simulink library "mylib"  (R2019b)
settings: Solver=VariableStepAuto  StartTime=0.0  StopTime=10.0  RelTol=1e-3
undefined symbols (not defined in the file or in its folder): AG, AH, AV, BCHL, BCHV, BG, BH, CG, CH, magnitude, Ts, XMW
libraries: $bdroot x28, TElib x2
(part 1 of 3)
settings Model: Creator=j3vos  LastModifiedBy=j3vos
settings DataIOCC: ReturnWorkspaceOutputs=off
settings DebuggingCC: ArithmeticOperatorsInVariantConditions=warning
settings SFSimCC: SimUseLocalCustomCode=off  CustomCodeUndefinedFunction=UseInterfaceOnly
settings RTWCC: RTWUseLocalCustomCode=off

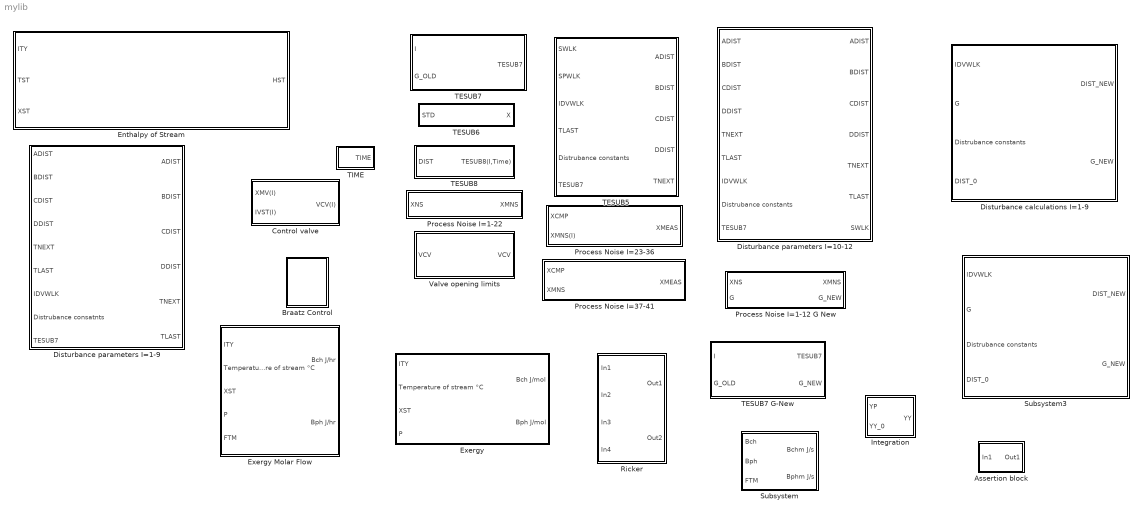
== system mylib ==
  Assertion block : Subsystem
      mask Display: color('Blue'),disp('Assertion\n Block')
  Braatz Control : Subsystem
  Control valve : Subsystem
      mask Display:
      | color('Green'), disp('Valve\nSticking');
      | color('Blue');
      | port_label('input',1,'XMV');
      | port_label('input',2,'IVST');
      | port_label('output',1,'VCV');
  Disturbance calculations I=1-9 : Subsystem
      mask Display:
      | color('Blue');
      | port_label('input',1,'IDVWLK');
      | port_label('input',2,'G');
      | port_label('input',3,'Disturbance constants');
      | port_label('input',4,'DIST_0');
      | port_label('output',1,'DIST_NEW');
      | port_label('output',2,'G_NEW');
      | color('Green'), disp('Disturbance Calculations\n I=1-9')
  Disturbance parameters I=1-9 : Subsystem
      mask Display:
      | color('Green'), disp('Disturbance parameters\n I=1-9');
      | color('Blue');
      | port_label('input',1,'ADIST');
      | port_label('input',2,'BDIST');
      | port_label('input',3,'CDIST');
      | port_label('input',4,'DDIST');
      | port_label('input',5,'TNEXT');
      | port_label('input',6,'TLAST');
      | port_label('input',7,'IDVWLK');
      | port_label('input',8,'Distrubance constants');
      | port_label('input',9,'TESUB7');
      | port_label('output',1,'ADIST');
      | port_label('output',2,'BDIST');
      | port_label('output',3,'CDIST');
      | port_label('output',4,'DDIST');
      | port_label('output',5,'TNEXT');
      | port_label('output',6,'TLAST');
  Disturbance parameters I=10-12 : Subsystem
      mask Display:
      | color('Green'), disp('Disturbance parameters\n I=10-12');
      | color('Blue');
      | port_label('input',1,'ADIST');
      | port_label('input',2,'BDIST');
      | port_label('input',3,'CDIST');
      | port_label('input',4,'DDIST');
      | port_label('input',5,'TNEXT');
      | port_label('input',6,'TLAST');
      | port_label('input',7,'IDVWLK');
      | port_label('input',8,'Distrubance constants');
      | port_label('input',9,'TESUB7');
      | port_label('output',1,'ADIST');
      | port_label('output',2,'BDIST');
      | port_label('output',3,'CDIST');
      | port_label('output',4,'DDIST');
      | port_label('output',5,'TNEXT');
      | port_label('output',6,'TLAST');
      | port_label('output',7,'SWLK');
  "Enthalpy of Stream " : Subsystem
      mask Display:
      | color('Green'), disp('TESUB1\nMolar Enthalpy of Stream\nMBtu/lb-mol');
      | color('Blue');
      | port_label('input',1,'Phase of Stream');
      | port_label('input',2,'Temperature of Stream');
      | port_label('input',3,'Composition of Stream');
      | port_label('output',1,'Enthalpy of Stream')
  Exergy : Subsystem
  Exergy Molar Flow : Subsystem
  Integration : Subsystem
  Process Noise I=1-12 G New : Subsystem
      mask Display:
      | color('Green'), disp('Process Noise');
      | color('Blue');
      | port_label('input',1,'XNS');
      | port_label('input',2,'G')
      | port_label('output',1,'XMNS');
      | port_label('output',2,'G_NEW')
  Process Noise I=1-22 : Subsystem
      mask Display:
      | color('Green'), disp('Process Noise\n I=1-22');
      | color('Blue');
      | port_label('input',1,'XNS');
      | port_label('output',1,'XMNS');
  Process Noise I=23-36 : Subsystem
      mask Display:
      | color('Green'), disp('Gas Analysis Delay\n I=23-36');
      | color('Blue');
      | port_label('input',1,'XCMP');
      | port_label('input',2,'XMNS');
      | port_label('output',1,'XMEAS');
  Process Noise I=37-41 : Subsystem
      mask Display:
      | color('Green'), disp('Product Analysis Delay\n I=37-41');
      | color('Blue');
      | port_label('input',1,'XCMP');
      | port_label('input',2,'XMNS');
      | port_label('output',1,'XMEAS');
  Ricker : Subsystem
  Subsystem : Subsystem
  Subsystem3 : Subsystem
      mask Display:
      | color('Blue');
      | port_label('input',1,'IDVWLK');
      | port_label('input',2,'G');
      | port_label('input',3,'Disturbance constants');
      | port_label('input',4,'DIST_0');
      | port_label('output',1,'DIST_NEW');
      | port_label('output',2,'G_NEW');
      | color('Green'), disp('Disturbance Calculations\n I=10-12')
  TESUB5 : Subsystem
      mask Display:
      | color('Green'), disp('TESUB5');
      | color('Blue');
      | port_label('input',1,'SWLK');
      | port_label('input',2,'SPWLK');
      | port_label('input',3,'IDVWLK');
      | port_label('input',4,'TLAST');
      | port_label('input',5,'Disturbance constants');
      | port_label('input',6,'TESUB7');
      | port_label('output',1,'ADIST');
      | port_label('output',2,'BDIST');
      | port_label('output',3,'CDIST');
      | port_label('output',4,'DDIST');
      | port_label('output',5,'TNEXT');
  TESUB6 : Subsystem
      mask Display:
      | color('Green'), disp('TESUB6');
      | color('Blue');
      | port_label('input',1,'XNS(I)');
      | port_label('output',1,'XMNS')
  TESUB7 : Subsystem
      mask Display:
      | color('Green'), port_label('output',1,'TESUB7');
      | color('Blue');
      | port_label('input',1,'I');
      | port_label('input',2,'Random number G');
  TESUB7 G-New : Subsystem
      mask Display:
      | color('Green'), port_label('output',1,'TESUB7');
      | color('Blue');
      | port_label('input',1,'I');
      | port_label('input',2,'Random number G');
  TESUB8 : Subsystem
      mask Display:
      | color('Blue');
      | port_label('input',1,'DIST');
      | color('Green'), port_label('output',1,'TESUB8(I,Time)')
  TIME : Subsystem
  Valve opening limits : Subsystem
      mask Display:
      | color('Green'), disp('Valve\nopening\nlimits');
      | color('Blue');
      | port_label('input',1,'VCV');
      | port_label('output',1,'VCV');

== system mylib/Assertion block ==
  In1 : Inport
  Data Type Conversion1 : DataTypeConversion  OutDataTypeStr=double
  Delay : Delay  DelayLength=1  InitialCondition=0
  If : If  NumInputs=2  IfExpression=u1 == 0  ElseIfExpressions=u2 == 1
  If Action Subsystem1 : Subsystem  TreatAsAtomicUnit=on
  If Action Subsystem2 : Subsystem  TreatAsAtomicUnit=on
  If Action Subsystem3 : Subsystem  TreatAsAtomicUnit=on
  Merge : Merge  Inputs=3
  Sum of Elements : Sum
  Out1 : Outport
  wires:
  If Action Subsystem2/1(Out1) -> Merge/3
  If Action Subsystem3/1(Out1) -> Merge/2
  If/1 -> If Action Subsystem1/Action
  Data Type Conversion1/1 -> Sum of Elements/1, If/1
  Sum of Elements/1 -> Delay/1, If/2
  If/3 -> If Action Subsystem2/Action
  If/2 -> If Action Subsystem3/Action
  If Action Subsystem1/1(Out1) -> Merge/1
  Delay/1 -> Sum of Elements/2
  In1/1 -> Data Type Conversion1/1
  Merge/1 -> Out1/1

== system mylib/Braatz Control ==
  P Control : Subsystem
  PI Control : Subsystem
  PI Control Setpoint : Subsystem
  Sampling interval : Subsystem
      mask Display: color('Blue'), disp('Sampling\ninterval');
  Subsystem1 : Subsystem
      mask Display: color('Blue'), disp('Valve open/close\nLimits');

== system mylib/Control valve ==
  XMV(I) : Inport
  IVST(I) : Inport  Port=2
  Delay : Delay  DelayLength=1  InitialConditionSource=Input port  InitialCondition=0
      settings: InputPortMap=u0,p4
  Subsystem : Subsystem
  Valve opening limits : $bdroot/Valve opening limits  SystemSampleTime=-1  Latency=0  AutoFrameSizeCalculation=off
  VCV(I) : Outport  VectorParamsAs1DForOutWhenUnconnected=off
  wires:
  Valve opening limits/1 -> Delay/1, VCV(I)/1
  XMV(I)/1 -> Subsystem/1(XMV(I)), Delay/2
  Delay/1 -> Subsystem/2("VCV(I) ")
  Subsystem/1(VCV(I)) -> Valve opening limits/1
  IVST(I)/1 -> Subsystem/3(IVST(I))

== system mylib/Disturbance calculations I=1-9 ==
  IDVWLK : Inport
  G : Inport  Port=2
  Distrubance constants : Inport  Port=3
  DIST_0 : Inport  Port=4
  Bus Selector : BusSelector  OutputSignals=TNEXT
  If Action Subsystem : Subsystem  TreatAsAtomicUnit=on
  If Action Subsystem1 : Subsystem  TreatAsAtomicUnit=on
  Merge : Merge
  Subsystem : Subsystem
  Subsystem1 : Subsystem
  Subsystem2 : Subsystem
  DIST_NEW : Outport  VectorParamsAs1DForOutWhenUnconnected=off
  G_NEW : Outport  Port=2  VectorParamsAs1DForOutWhenUnconnected=off
  wires:
  Subsystem2/1(G1) -> G_NEW/1
  If Action Subsystem/1(DIST_NEW) -> Merge/2
  Bus Selector/1 -> Subsystem/1(TNEXT)  "<TNEXT>"
  If Action Subsystem1/1(DIST) -> Merge/1
  DIST_0/1 -> If Action Subsystem1/1(DIST_0)
  Merge/1 -> Subsystem1/1(DIST_NEW), DIST_NEW/1
  IDVWLK/1 -> If Action Subsystem/1(IDVWLK)
  G/1 -> Subsystem2/2(G), If Action Subsystem/3(G)
  Distrubance constants/1 -> If Action Subsystem/4(Distrubance constants)
  Subsystem1/1(DIST) -> If Action Subsystem/2("DIST "), Bus Selector/1
  If Action Subsystem/2(G_NEW) -> Subsystem2/1(In2)
  Subsystem/1(if) -> If Action Subsystem1/Action
  Subsystem/2(elseif) -> If Action Subsystem/Action

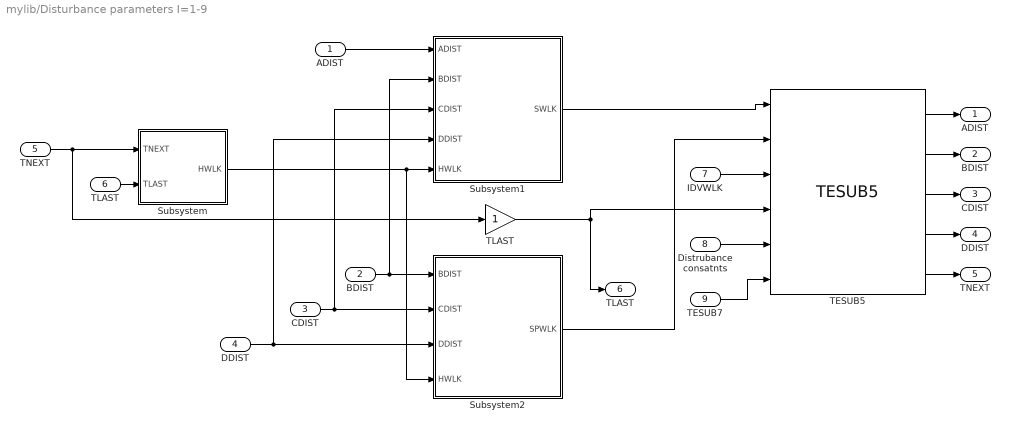
== system mylib/Disturbance parameters I=1-9 ==
  ADIST : Inport
  BDIST : Inport  Port=2
  CDIST : Inport  Port=3
  DDIST : Inport  Port=4
  TNEXT : Inport  Port=5
  TLAST : Inport  Port=6
  IDVWLK : Inport  Port=7
  Distrubance consatnts : Inport  Port=8
  TESUB7 : Inport  Port=9
  Subsystem : Subsystem
  Subsystem1 : Subsystem
  Subsystem2 : Subsystem
  TESUB5 : $bdroot/TESUB5  SystemSampleTime=-1  Latency=0  AutoFrameSizeCalculation=off
  "TLAST " : Gain
  "ADIST " : Outport  VectorParamsAs1DForOutWhenUnconnected=off
  "BDIST " : Outport  Port=2  VectorParamsAs1DForOutWhenUnconnected=off
  "CDIST " : Outport  Port=3  VectorParamsAs1DForOutWhenUnconnected=off
  "DDIST " : Outport  Port=4  VectorParamsAs1DForOutWhenUnconnected=off
  "TNEXT " : Outport  Port=5  VectorParamsAs1DForOutWhenUnconnected=off
  "TLAST  " : Outport  Port=6  VectorParamsAs1DForOutWhenUnconnected=off
  wires:
  BDIST/1 -> Subsystem2/1(BDIST), Subsystem1/2(BDIST)
  CDIST/1 -> Subsystem1/3(CDIST), Subsystem2/2(CDIST)
  DDIST/1 -> Subsystem1/4(DDIST), Subsystem2/3(DDIST)
  IDVWLK/1 -> TESUB5/3
  TNEXT/1 -> "TLAST "/1, Subsystem/1(TNEXT)
  "TLAST "/1 -> TESUB5/4, "TLAST  "/1
  TESUB5/1 -> "ADIST "/1
  TESUB5/2 -> "BDIST "/1
  TESUB5/3 -> "CDIST "/1
  TESUB5/4 -> "DDIST "/1
  TESUB5/5 -> "TNEXT "/1
  TLAST/1 -> Subsystem/2(TLAST)
  ADIST/1 -> Subsystem1/1(ADIST)
  Subsystem1/1("SWLK ") -> TESUB5/1
  Subsystem/1("HWLK ") -> Subsystem2/4(HWLK), Subsystem1/5(HWLK)
  Subsystem2/1("SPWLK ") -> TESUB5/2
  Distrubance consatnts/1 -> TESUB5/5
  TESUB7/1 -> TESUB5/6

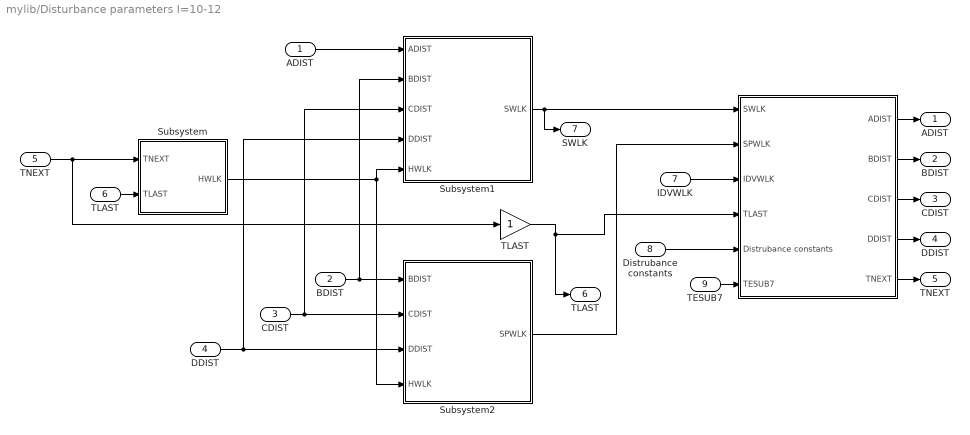
== system mylib/Disturbance parameters I=10-12 ==
  ADIST : Inport
  BDIST : Inport  Port=2
  CDIST : Inport  Port=3
  DDIST : Inport  Port=4
  TNEXT : Inport  Port=5
  TLAST : Inport  Port=6
  IDVWLK : Inport  Port=7
  Distrubance constants : Inport  Port=8
  TESUB7 : Inport  Port=9
  " " : Subsystem
  Subsystem : Subsystem
  Subsystem1 : Subsystem
  Subsystem2 : Subsystem
  "TLAST " : Gain
  "ADIST " : Outport  VectorParamsAs1DForOutWhenUnconnected=off
  "BDIST " : Outport  Port=2  VectorParamsAs1DForOutWhenUnconnected=off
  "CDIST " : Outport  Port=3  VectorParamsAs1DForOutWhenUnconnected=off
  "DDIST " : Outport  Port=4  VectorParamsAs1DForOutWhenUnconnected=off
  "TNEXT " : Outport  Port=5  VectorParamsAs1DForOutWhenUnconnected=off
  "TLAST  " : Outport  Port=6  VectorParamsAs1DForOutWhenUnconnected=off
  SWLK : Outport  Port=7  VectorParamsAs1DForOutWhenUnconnected=off
  wires:
  BDIST/1 -> Subsystem2/1(BDIST), Subsystem1/2(BDIST)
  CDIST/1 -> Subsystem1/3(CDIST), Subsystem2/2(CDIST)
  DDIST/1 -> Subsystem1/4(DDIST), Subsystem2/3(DDIST)
  IDVWLK/1 -> " "/3(IDVWLK)
  TNEXT/1 -> "TLAST "/1, Subsystem/1(TNEXT)
  "TLAST "/1 -> "TLAST  "/1, " "/4(TLAST)
  " "/1(ADIST) -> "ADIST "/1
  " "/2(BDIST) -> "BDIST "/1
  " "/3(CDIST) -> "CDIST "/1
  " "/4(DDIST) -> "DDIST "/1
  " "/5(TNEXT) -> "TNEXT "/1
  TLAST/1 -> Subsystem/2(TLAST)
  ADIST/1 -> Subsystem1/1(ADIST)
  Subsystem1/1("SWLK ") -> SWLK/1, " "/1(SWLK)
  Subsystem/1("HWLK ") -> Subsystem1/5(HWLK), Subsystem2/4(HWLK)
  Subsystem2/1("SPWLK ") -> " "/2(SPWLK)
  Distrubance constants/1 -> " "/5(Distrubance constants)
  TESUB7/1 -> " "/6(TESUB7)

== system mylib/Enthalpy of Stream  ==
  ITY : Inport
  TST : Inport  Port=2
  XST : Inport  Port=3
  Calculate Enthalpy if ITY=2 : Subsystem
  Calculate Molar Liquid Enthalpy of stream MBtu/lb-mol : Subsystem
  Calculate Molar Vapour Enthalpy of stream MBtu/lb-mol : Subsystem
  H Molar Enthalpy of stream MBtu/lb-mol : Merge  Inputs=3
  If : If  IfExpression=u1 == 0  ElseIfExpressions=u1 == 2
  If Action Subsystem : Subsystem  TreatAsAtomicUnit=on
  If Action Subsystem1 : Subsystem  TreatAsAtomicUnit=on
  If Action Subsystem2 : Subsystem  TreatAsAtomicUnit=on
  HST : Outport  VectorParamsAs1DForOutWhenUnconnected=off
  wires:
  Calculate Molar Vapour Enthalpy of stream MBtu/lb-mol/1(H) -> Calculate Enthalpy if ITY=2/2(H), If Action Subsystem2/1(In1)
  If/2 -> If Action Subsystem1/Action
  TST/1 -> Calculate Molar Liquid Enthalpy of stream MBtu/lb-mol/1(T), Calculate Enthalpy if ITY=2/1(T), Calculate Molar Vapour Enthalpy of stream MBtu/lb-mol/1(T)
  XST/1 -> Calculate Molar Vapour Enthalpy of stream MBtu/lb-mol/2(XST(I,1)), Calculate Molar Liquid Enthalpy of stream MBtu/lb-mol/2(XST(I,1))
  If Action Subsystem1/1(Out1) -> H Molar Enthalpy of stream MBtu/lb-mol/2
  If/1 -> If Action Subsystem/Action
  Calculate Enthalpy if ITY=2/1("H ") -> If Action Subsystem1/1(In1)
  ITY/1 -> If/1
  Calculate Molar Liquid Enthalpy of stream MBtu/lb-mol/1(H) -> If Action Subsystem/1(In1)
  If Action Subsystem2/1(Out1) -> H Molar Enthalpy of stream MBtu/lb-mol/3
  If/3 -> If Action Subsystem2/Action
  If Action Subsystem/1(Out1) -> H Molar Enthalpy of stream MBtu/lb-mol/1
  H Molar Enthalpy of stream MBtu/lb-mol/1 -> HST/1

== system mylib/Exergy ==
  ITY : Inport
  Temperature of stream °C : Inport  Port=2
  XST : Inport  Port=3
  P : Inport  Port=4
  Gain : Gain  Gain=2.32601*10e6
  Subsystem : Subsystem
  Subsystem2 : Subsystem
  Bch J/mol : Outport  VectorParamsAs1DForOutWhenUnconnected=off
  Bph J/mol : Outport  Port=2  VectorParamsAs1DForOutWhenUnconnected=off
  wires:
  ITY/1 -> Subsystem/1(ITY), Subsystem2/1(ITY)
  Temperature of stream °C/1 -> Subsystem2/2(Temperature of stream °C)
  XST/1 -> Subsystem/2("XST "), Subsystem2/3(XST)
  P/1 -> Subsystem2/4(P)
  Subsystem2/1(Bph MBtu/lb-mol) -> Gain/1
  Subsystem/1(Bch J/mol) -> Bch J/mol/1
  Gain/1 -> Bph J/mol/1

== system mylib/Exergy Molar Flow ==
  ITY : Inport
  Temperature of stream °C : Inport  Port=2
  XST : Inport  Port=3
  P : Inport  Port=4
  FTM : Inport  Port=5
  Gain : Gain  Gain=2.32601*10e6
  Product : Product
  Product1 : Product
  Subsystem : Subsystem
  Subsystem2 : Subsystem
  mol : Constant  Value=453.59
  mol/h : Product
  Bch J/hr : Outport  VectorParamsAs1DForOutWhenUnconnected=off
  Bph J/hr : Outport  Port=2  VectorParamsAs1DForOutWhenUnconnected=off
  wires:
  Subsystem2/1(Bph MBtu/lb-mol) -> Gain/1
  P/1 -> Subsystem2/4(P)
  XST/1 -> Subsystem2/3(XST), Subsystem/2("XST ")
  Temperature of stream °C/1 -> Subsystem2/2(Temperature of stream °C)
  ITY/1 -> Subsystem2/1(ITY), Subsystem/1(ITY)
  mol/1 -> mol/h/1
  FTM/1 -> mol/h/2
  mol/h/1 -> Product1/2, Product/2
  Subsystem/1(Bch kJ/mol) -> Product/1
  Product/1 -> Bch J/hr/1
  Gain/1 -> Product1/1
  Product1/1 -> Bph J/hr/1

== system mylib/Integration ==
  YP : Inport
  YY_0 : Inport  Port=2
  Display{,1..3} (4 alike) : Display
  Integrator : Integrator  InitialConditionSource=external
  Subsystem : Subsystem
  YY : Outport
  wires:
  YY_0/1 -> Integrator/2, Display3/1
  Integrator/1 -> YY/1, Display/1
  YP/1 -> Subsystem/1(In1), Display2/1
  Subsystem/1(Out1) -> Integrator/1, Display1/1

== system mylib/Process Noise I=1-12 G New ==
  XNS : Inport
  G : Inport  Port=2
  TESUB6 : Subsystem
      mask Display:
      | color('Green'), disp('TESUB6');
      | color('Blue');
      | port_label('input',1,'XNS(I)');
      | port_label('input',2,'G');
      | port_label('output',1,'XMNS');
      | port_label('output',2,'G_NEW')
  XMNS : Outport  VectorParamsAs1DForOutWhenUnconnected=off
  G_NEW : Outport  Port=2  VectorParamsAs1DForOutWhenUnconnected=off
  wires:
  XNS/1 -> TESUB6/1(STD)
  TESUB6/1(X) -> XMNS/1
  TESUB6/2(G_NEW) -> G_NEW/1
  G/1 -> TESUB6/2(G)

== system mylib/Process Noise I=1-22 ==
  XNS : Inport
  Clock : Clock
  If : If  NumInputs=2  IfExpression=u1>0 & u2==1  ShowElse=off
  If Action Subsystem : Subsystem  TreatAsAtomicUnit=on
  TESUB6 : $bdroot/TESUB6  SystemSampleTime=-1  Latency=0  AutoFrameSizeCalculation=off
  XMNS : Outport  VectorParamsAs1DForOutWhenUnconnected=off
  wires:
  [ISD] -> If/2
  If/1 -> If Action Subsystem/Action
  XNS/1 -> TESUB6/1
  Clock/1 -> If/1
  TESUB6/1 -> If Action Subsystem/1(In1)
  If Action Subsystem/1(Out1) -> XMNS/1

== system mylib/Process Noise I=23-36 ==
  XCMP : Inport
  XMNS(I) : Inport  Port=2
  Clock : Clock
  Delay : Delay  DelayLength=1  InitialConditionSource=Input port  InitialCondition=0
      settings: InputPortMap=u0,p4
  Delay1 : Delay  DelayLength=1  InitialConditionSource=Input port  InitialCondition=0
      settings: InputPortMap=u0,p4
  Gas Analysis Delay : Subsystem
  If : If  IfExpression=u1 == 0  ShowElse=off
  If Action Subsystem : Subsystem  TreatAsAtomicUnit=on
  If Action Subsystem1 : Subsystem  TreatAsAtomicUnit=on
  XMEAS : Outport  VectorParamsAs1DForOutWhenUnconnected=off
  wires:
  Delay1/1 -> XMEAS/1
  If/1 -> If Action Subsystem1/Action
  Clock/1 -> If/1
  Delay/1 -> If Action Subsystem/2(XDEL_OLD)
  If Action Subsystem1/1(Out1) -> Delay/2
  Gas Analysis Delay/1(IF(TGAS)) -> If Action Subsystem/Action
  If Action Subsystem/1(XDEL_NEW) -> Delay/1
  If Action Subsystem/2(XMEAS) -> Delay1/1
  XCMP/1 -> If Action Subsystem1/1(In1), If Action Subsystem/1(XCMP), Delay1/2
  XMNS(I)/1 -> If Action Subsystem/3(XMNS)

== system mylib/Process Noise I=37-41 ==
  XCMP : Inport
  XMNS : Inport  Port=2
  Clock : Clock
  Delay : Delay  DelayLength=1  InitialConditionSource=Input port  InitialCondition=0
      settings: InputPortMap=u0,p4
  Delay1 : Delay  DelayLength=1  InitialConditionSource=Input port  InitialCondition=0
      settings: InputPortMap=u0,p4
  Gas Analysis Delay : Subsystem
  If : If  IfExpression=u1 == 0  ShowElse=off
  If Action Subsystem : Subsystem  TreatAsAtomicUnit=on
  If Action Subsystem1 : $bdroot/Process Noise I=23-36/If Action Subsystem1  SystemSampleTime=-1  Latency=0  AutoFrameSizeCalculation=off
  XMEAS : Outport  VectorParamsAs1DForOutWhenUnconnected=off
  wires:
  Delay1/1 -> XMEAS/1
  XCMP/1 -> If Action Subsystem1/1, If Action Subsystem/1(XCMP), Delay1/2
  XMNS/1 -> If Action Subsystem/3(XMNS)
  Delay/1 -> If Action Subsystem/2(XDEL_OLD)
  If Action Subsystem/1(XDEL_NEW) -> Delay/1
  If/1 -> If Action Subsystem1/Action
  Gas Analysis Delay/1(IF(TPROD)) -> If Action Subsystem/Action
  If Action Subsystem1/1 -> Delay/2
  If Action Subsystem/2(XMEAS) -> Delay1/1
  Clock/1 -> If/1

== system mylib/Ricker ==
  In1 : Inport
  In2 : Inport  Port=2
  In3 : Inport  Port=3
  In4 : Inport  Port=4
  Discrete PI : TElib/Discrete PI  Kc=0  Ti=inf  Ts=1  x0=0  Hi=1  Lo=-1
  Vel PI : TElib/Discrete PI/Vel PI  Kc=Kc  Ti=Ti  Ts=Ts
  Out1 : Outport  VectorParamsAs1DForOutWhenUnconnected=off
  Out2 : Outport  Port=2  VectorParamsAs1DForOutWhenUnconnected=off
  wires:
  In3/1 -> Vel PI/1
  In1/1 -> Discrete PI/1
  In4/1 -> Vel PI/2
  Vel PI/1 -> Out2/1
  In2/1 -> Discrete PI/2
  Discrete PI/1 -> Out1/1

== system mylib/Subsystem ==
  Bch : Inport
  Bph : Inport  Port=2
  FTM : Inport  Port=3
  Gain : Gain  Gain=1/3600
  Gain1 : Gain  Gain=1/3600
  Product : Product
  Product1 : Product
  mol : Constant  Value=453.59
  mol/h : Product
  Bchm J/s : Outport  VectorParamsAs1DForOutWhenUnconnected=off
  Bphm J/s : Outport  Port=2  VectorParamsAs1DForOutWhenUnconnected=off
  wires:
  Gain1/1 -> Bchm J/s/1
  Gain/1 -> Bphm J/s/1
  Bch/1 -> Product/1
  mol/h/1 -> Product/2, Product1/2
  FTM/1 -> mol/h/2
  mol/1 -> mol/h/1
  Product1/1 -> Gain/1
  Product/1 -> Gain1/1
  Bph/1 -> Product1/1

== system mylib/Subsystem3 ==
  IDVWLK : Inport
  G : Inport  Port=2
  Distrubance constants : Inport  Port=3
  DIST_0 : Inport  Port=4
  Bus Selector : BusSelector  OutputSignals=TNEXT
  If Action Subsystem : Subsystem  TreatAsAtomicUnit=on
  If Action Subsystem1 : Subsystem  TreatAsAtomicUnit=on
  Merge : Merge
  Subsystem : Subsystem
  Subsystem1 : Subsystem
  Subsystem2 : Subsystem
  DIST_NEW : Outport  VectorParamsAs1DForOutWhenUnconnected=off
  G_NEW : Outport  Port=2  VectorParamsAs1DForOutWhenUnconnected=off
  wires:
  If Action Subsystem/1(DIST_NEW) -> Merge/2
  IDVWLK/1 -> If Action Subsystem/1(IDWLK)
  If Action Subsystem1/1(DIST) -> Merge/1
  Subsystem1/1(DIST) -> If Action Subsystem/2("DIST "), Bus Selector/1
  Merge/1 -> Subsystem1/1(DIST_NEW), DIST_NEW/1
  G/1 -> Subsystem2/2(G), If Action Subsystem/3(G)
  If Action Subsystem/2("G_NEW ") -> Subsystem2/1(In2)
  Subsystem2/1(G1) -> G_NEW/1
  Distrubance constants/1 -> If Action Subsystem/4(Distrubance constants)
  DIST_0/1 -> If Action Subsystem1/1(DIST_0)
  Bus Selector/1 -> Subsystem/1(TNEXT)  "<TNEXT>"
  Subsystem/1(if) -> If Action Subsystem1/Action
  Subsystem/2(elseif) -> If Action Subsystem/Action

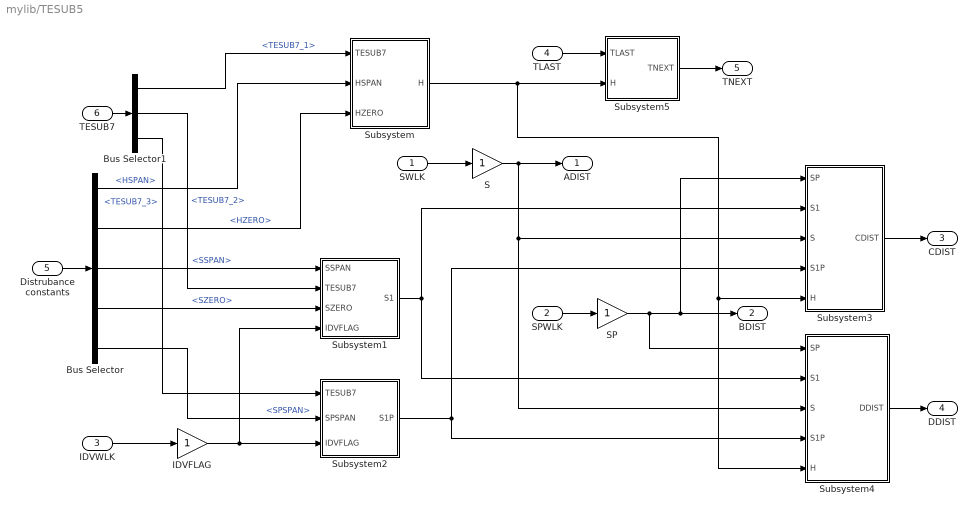
== system mylib/TESUB5 ==
  SWLK : Inport
  SPWLK : Inport  Port=2
  IDVWLK : Inport  Port=3
  TLAST : Inport  Port=4
  "Distrubance constants " : Inport  Port=5
  TESUB7 : Inport  Port=6
  Bus Selector : BusSelector  OutputSignals=HSPAN,HZERO,SSPAN,SZERO,SPSPAN
  Bus Selector1 : BusSelector  OutputSignals=TESUB7_1,TESUB7_2,TESUB7_3
  IDVFLAG : Gain
  S : Gain
  SP : Gain
  Subsystem : Subsystem
  Subsystem1 : Subsystem
  Subsystem2 : Subsystem
  Subsystem3 : Subsystem
  Subsystem4 : Subsystem
  Subsystem5 : Subsystem
  ADIST : Outport  VectorParamsAs1DForOutWhenUnconnected=off
  BDIST : Outport  Port=2  VectorParamsAs1DForOutWhenUnconnected=off
  CDIST : Outport  Port=3  VectorParamsAs1DForOutWhenUnconnected=off
  DDIST : Outport  Port=4  VectorParamsAs1DForOutWhenUnconnected=off
  TNEXT : Outport  Port=5  VectorParamsAs1DForOutWhenUnconnected=off
  wires:
  Bus Selector1/3 -> Subsystem2/1(TESUB7)  "<TESUB7_3>"
  Bus Selector1/2 -> Subsystem1/2(TESUB7)  "<TESUB7_2>"
  Bus Selector1/1 -> Subsystem/1(TESUB7)  "<TESUB7_1>"
  TESUB7/1 -> Bus Selector1/1
  IDVWLK/1 -> IDVFLAG/1
  IDVFLAG/1 -> Subsystem1/4(IDVFLAG), Subsystem2/3(IDVFLAG)
  SWLK/1 -> S/1
  SPWLK/1 -> SP/1
  S/1 -> ADIST/1, Subsystem4/3(S), Subsystem3/3(S)
  SP/1 -> Subsystem3/1(SP), BDIST/1, Subsystem4/1(SP)
  Subsystem/1("H ") -> Subsystem5/2(H), Subsystem4/5(H), Subsystem3/5(H)
  Subsystem1/1("S1 ") -> Subsystem3/2(S1), Subsystem4/2(S1)
  Subsystem2/1("S1P ") -> Subsystem3/4(S1P), Subsystem4/4(S1P)
  Subsystem3/1(CDIST) -> CDIST/1
  Subsystem4/1(DDIST) -> DDIST/1
  TLAST/1 -> Subsystem5/1(TLAST)
  Subsystem5/1(TNEXT) -> TNEXT/1
  Bus Selector/4 -> Subsystem1/3(SZERO)  "<SZERO>"
  Bus Selector/3 -> Subsystem1/1(SSPAN)  "<SSPAN>"
  Bus Selector/1 -> Subsystem/2(HSPAN)  "<HSPAN>"
  Bus Selector/5 -> Subsystem2/2(SPSPAN)  "<SPSPAN>"
  "Distrubance constants "/1 -> Bus Selector/1
  Bus Selector/2 -> Subsystem/3(HZERO)  "<HZERO>"

== system mylib/TESUB6 ==
  STD : Inport
  Constant : Constant  Value=6
  I : Constant  Value=1:12
  Product : Product
  Subtract : Sum  Inputs=+-
  TESUB7 : Subsystem
  X : Outport  VectorParamsAs1DForOutWhenUnconnected=off
  wires:
  I/1 -> TESUB7/2(I)
  [G] -> TESUB7/1(G)
  TESUB7/1(TESUB7) -> Subtract/1
  Constant/1 -> Subtract/2
  Subtract/1 -> Product/1
  Product/1 -> X/1
  STD/1 -> Product/2

== system mylib/TESUB7 ==
  I : Inport
  G_OLD : Inport  Port=2
  Constant : Constant  Value=2
  Constant1 : Constant  Value=4294967296
  Constant2 : Constant
  Divide : Product  Inputs=*/
  Divide1 : Product  Inputs=**/
  Gain : Gain  Gain=9228907
  If : If  IfExpression=u1 >=0  ElseIfExpressions=u1 <0  ShowElse=off
  If Action Subsystem : Subsystem  TreatAsAtomicUnit=on
  If Action Subsystem1 : Subsystem  TreatAsAtomicUnit=on
  Merge1 : Merge
  New G : Math  Operator=rem  SaturateOnIntegerOverflow=on
  Subtract : Sum  Inputs=+-
  TESUB7 : Outport  VectorParamsAs1DForOutWhenUnconnected=off
  wires:
  Divide/1 -> If Action Subsystem/1(In1)
  I/1 -> If/1
  If/1 -> If Action Subsystem/Action
  If/2 -> If Action Subsystem1/Action
  G_OLD/1 -> Gain/1
  Gain/1 -> New G/1
  Constant1/1 -> Divide1/3, Divide/2, New G/2
  New G/1 -> Divide/1, Divide1/2
  Constant/1 -> Divide1/1
  Divide1/1 -> Subtract/1
  Constant2/1 -> Subtract/2
  Subtract/1 -> If Action Subsystem1/1(In1)
  Merge1/1 -> TESUB7/1
  If Action Subsystem/1(Out1) -> Merge1/1
  If Action Subsystem1/1(Out1) -> Merge1/2

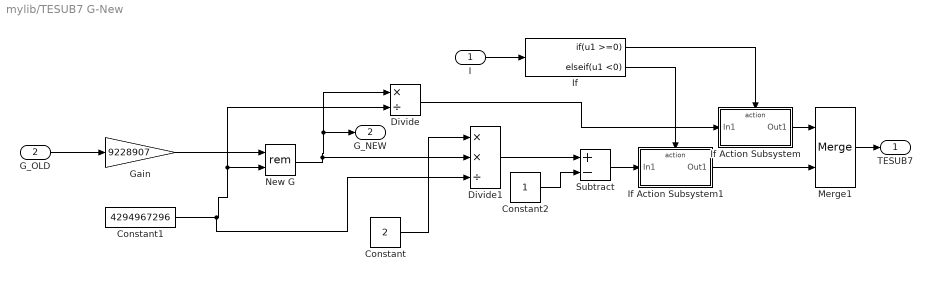
== system mylib/TESUB7 G-New ==
  I : Inport
  G_OLD : Inport  Port=2
  Constant : Constant  Value=2
  Constant1 : Constant  Value=4294967296
  Constant2 : Constant
  Divide : Product  Inputs=*/
  Divide1 : Product  Inputs=**/
  Gain : Gain  Gain=9228907
  If : If  IfExpression=u1 >=0  ElseIfExpressions=u1 <0  ShowElse=off
  If Action Subsystem : Subsystem  TreatAsAtomicUnit=on
  If Action Subsystem1 : Subsystem  TreatAsAtomicUnit=on
  Merge1 : Merge
  New G : Math  Operator=rem  SaturateOnIntegerOverflow=on
  Subtract : Sum  Inputs=+-
  TESUB7 : Outport  VectorParamsAs1DForOutWhenUnconnected=off
  G_NEW : Outport  Port=2  VectorParamsAs1DForOutWhenUnconnected=off
  wires:
  Divide/1 -> If Action Subsystem/1(In1)
  I/1 -> If/1
  If/1 -> If Action Subsystem/Action
  If/2 -> If Action Subsystem1/Action
  G_OLD/1 -> Gain/1
  Gain/1 -> New G/1
  Constant1/1 -> Divide1/3, Divide/2, New G/2
  New G/1 -> G_NEW/1, Divide/1, Divide1/2
  Constant/1 -> Divide1/1
  Divide1/1 -> Subtract/1
  Constant2/1 -> Subtract/2
  Subtract/1 -> If Action Subsystem1/1(In1)
  Merge1/1 -> TESUB7/1
  If Action Subsystem/1(Out1) -> Merge1/1
  If Action Subsystem1/1(Out1) -> Merge1/2

== system mylib/TESUB8 ==
  DIST : Inport
  Add : Sum
  Add1 : Sum
  Add2 : Sum
  Bus Selector : BusSelector  OutputSignals=ADIST,BDIST,CDIST,DDIST,TLAST
  H : Sum  Inputs=+-
  Product : Product
  Product1 : Product
  Product2 : Product
  Time : Clock
  TESUB8(I,Time) : Outport  PortDimensions=1  VectorParamsAs1DForOutWhenUnconnected=off
  wires:
  Add2/1 -> Product1/1
  H/1 -> Product/2, Product1/2, Product2/2
  Time/1 -> H/1
  Add1/1 -> Product/1
  Product2/1 -> Add2/2
  Add/1 -> TESUB8(I,Time)/1
  Product/1 -> Add/2
  Product1/1 -> Add1/2
  Bus Selector/2 -> Add1/1  "<BDIST>"
  Bus Selector/5 -> H/2  "<TLAST>"
  Bus Selector/4 -> Product2/1  "<DDIST>"
  DIST/1 -> Bus Selector/1
  Bus Selector/1 -> Add/1  "<ADIST>"
  Bus Selector/3 -> Add2/1  "<CDIST>"

== system mylib/TIME ==
  Add : Sum
  Delay : Delay  DelayLength=1  InitialConditionSource=Input port  InitialCondition=0
      settings: InputPortMap=u0,p4
  Deltat : Constant  Value=1/3600
  TIME_0 : Constant  Value=0
  TIME : Outport
  wires:
  TIME_0/1 -> Delay/2
  Add/1 -> Delay/1
  Delay/1 -> TIME/1, Add/1
  Deltat/1 -> Add/2

== system mylib/Valve opening limits ==
  VCV : Inport
  Abs : Abs
  Constant : Constant  Value=0
  Constant1 : Constant  Value=100
  If : If  IfExpression=u1 < 0  ElseIfExpressions=u1>100
  If Action Subsystem : Subsystem  TreatAsAtomicUnit=on
  If Action Subsystem1 : Subsystem  TreatAsAtomicUnit=on
  If Action Subsystem2 : Subsystem  TreatAsAtomicUnit=on
  Merge1 : Merge  Inputs=3
  "VCV " : Outport  VectorParamsAs1DForOutWhenUnconnected=off
  wires:
  If/3 -> If Action Subsystem2/Action
  If Action Subsystem/1(Out1) -> Merge1/1
  Constant/1 -> If Action Subsystem/1(In1)
  VCV/1 -> If/1, If Action Subsystem2/1(In1)
  If/2 -> If Action Subsystem1/Action
  If Action Subsystem2/1(Out1) -> Merge1/2
  If/1 -> If Action Subsystem/Action
  Abs/1 -> "VCV "/1
  Constant1/1 -> If Action Subsystem1/1(In1)
  Merge1/1 -> Abs/1
  If Action Subsystem1/1(Out1) -> Merge1/3

== system mylib/Assertion block/If Action Subsystem1 ==
  Action Port : ActionPort
  Constant : Constant
  Out1 : Outport
  wires:
  Constant/1 -> Out1/1

== system mylib/Assertion block/If Action Subsystem2 ==
  Action Port : ActionPort
  Constant : Constant
  Out1 : Outport
  wires:
  Constant/1 -> Out1/1

== system mylib/Assertion block/If Action Subsystem3 ==
  Action Port : ActionPort
  Constant : Constant  Value=0
  Out1 : Outport
  wires:
  Constant/1 -> Out1/1

== system mylib/Braatz Control/P Control ==
  SETPT : Inport
  GAIN : Inport  Port=2
  XMEAS : Inport  Port=3
  High Limit : Inport  Port=4
  XMV_0 : Inport  Port=5
  Action Port : ActionPort
  " " : Subsystem
  Delay1 : Delay  DelayLength=1  InitialConditionSource=Input port  InitialCondition=0
      settings: InputPortMap=u0,p4
  ERR : Subsystem
  ERROLD : Constant  Value=0
  Subsystem : Subsystem
  XMV_NEW : Outport  VectorParamsAs1DForOutWhenUnconnected=off
  wires:
  Delay1/1 -> Subsystem/3(ERROLD)
  XMV_0/1 -> " "/2(XMV_0)
  ERROLD/1 -> Delay1/2
  SETPT/1 -> ERR/1(SETPT)
  " "/1(XMV) -> XMV_NEW/1
  XMEAS/1 -> ERR/2(XMEAS)
  High Limit/1 -> ERR/3(High Limit)
  GAIN/1 -> Subsystem/2(GAIN)
  Subsystem/1(DXMV) -> " "/1(DXMV)  "DXMV"
  ERR/1(ERR) -> Subsystem/1(ERR), Delay1/1

== system mylib/Braatz Control/PI Control ==
  SETPT : Inport
  XMEAS : Inport  Port=2
  High Limit : Inport  Port=3
  GAIN : Inport  Port=4
  Sampling Interval : Inport  Port=5
  TAUI : Inport  Port=6
  XMV_0 : Inport  Port=7
  Action Port : ActionPort
  " " : $bdroot/Braatz Control/P Control/   SystemSampleTime=-1  Latency=0  AutoFrameSizeCalculation=off
  Delay1 : Delay  DelayLength=1  InitialConditionSource=Input port  InitialCondition=0
      settings: InputPortMap=u0,p4
  ERR : Subsystem
  ERROLD : Constant  Value=0
  Subsystem : Subsystem
  XMV_NEW : Outport  VectorParamsAs1DForOutWhenUnconnected=off
  wires:
  ERROLD/1 -> Delay1/2
  ERR/1(ERR) -> Delay1/1, Subsystem/1(ERR)
  SETPT/1 -> ERR/1(SETPT)
  Subsystem/1(DXMV) -> " "/1  "DXMV"
  " "/1 -> XMV_NEW/1
  XMEAS/1 -> ERR/2(XMEAS)
  High Limit/1 -> ERR/3(High Limit)
  GAIN/1 -> Subsystem/2(GAIN)
  Sampling Interval/1 -> Subsystem/3(Sampling Interval)
  TAUI/1 -> Subsystem/4(TAUI)
  Delay1/1 -> Subsystem/5(ERROLD)
  XMV_0/1 -> " "/2

== system mylib/Braatz Control/PI Control Setpoint ==
  SETPT : Inport
  XMEAS : Inport  Port=2
  High Limit Setpoint : Inport  Port=3
  High Limit : Inport  Port=4
  GAIN : Inport  Port=5
  Sampling Interval : Inport  Port=6
  TAUI : Inport  Port=7
  SETPT_0 : Inport  Port=8
  Action Port : ActionPort
  " " : Subsystem
  Delay1 : Delay  DelayLength=1  InitialConditionSource=Input port  InitialCondition=0
      settings: InputPortMap=u0,p4
  ERR : Subsystem
  ERROLD : Constant  Value=0
  Subsystem2 : Subsystem
  SETPT_NEW : Outport  VectorParamsAs1DForOutWhenUnconnected=off
  wires:
  SETPT_0/1 -> " "/3(SETPT_0)
  " "/1(SETPT) -> SETPT_NEW/1
  ERROLD/1 -> Delay1/2
  Delay1/1 -> Subsystem2/5(ERROLD)
  ERR/1(ERR) -> Subsystem2/1(ERR), Delay1/1
  High Limit/1 -> " "/2(High Limit)
  Subsystem2/1(DXMV) -> " "/1(DXMV)
  SETPT/1 -> ERR/1(SETPT)
  XMEAS/1 -> ERR/2(XMEAS)
  GAIN/1 -> Subsystem2/2(GAIN)
  Sampling Interval/1 -> Subsystem2/3(Sampling Interval)
  TAUI/1 -> Subsystem2/4(TAUI)
  High Limit Setpoint/1 -> ERR/3(High Limit Setpoint)

== system mylib/Braatz Control/Sampling interval ==
  Sampling interval number : Inport
  Clock : Clock
  Constant1 : Constant  Value=3600
  If1 : If  IfExpression=u1 == 0  ShowElse=off
  Math Function : Math  Operator=mod  SaturateOnIntegerOverflow=on
  Merge : Merge
  Product : Product
  Subsystem : Subsystem
      mask Display: color('Blue'), disp('MOD\nFix');
  TEST : Outport  VectorParamsAs1DForOutWhenUnconnected=off
  wires:
  If1/1 -> TEST/1
  Clock/1 -> Product/1
  Constant1/1 -> Product/2
  Sampling interval number/1 -> Subsystem/2(In2), Math Function/2
  Product/1 -> Math Function/1
  Merge/1 -> If1/1
  Math Function/1 -> Subsystem/1(In1)
  Subsystem/1(Out1) -> Merge/1
  Subsystem/2(Out2) -> Merge/2

== system mylib/Braatz Control/Subsystem1 ==
  XMV : Inport
  Constant : Constant  Value=0
  Constant1 : Constant  Value=100
  If : If  IfExpression=u1 < 0  ElseIfExpressions=u1 > 100
  If Action Subsystem : Subsystem  TreatAsAtomicUnit=on
  If Action Subsystem1 : Subsystem  TreatAsAtomicUnit=on
  If Action Subsystem2 : Subsystem  TreatAsAtomicUnit=on
  Merge : Merge  Inputs=3
  "XMV " : Outport  VectorParamsAs1DForOutWhenUnconnected=off
  wires:
  If Action Subsystem1/1(Out1) -> Merge/2
  If/1 -> If Action Subsystem/Action
  Merge/1 -> "XMV "/1
  Constant1/1 -> If Action Subsystem1/1(In1)
  If Action Subsystem2/1(Out1) -> Merge/3
  If/2 -> If Action Subsystem1/Action
  If/3 -> If Action Subsystem2/Action
  If Action Subsystem/1(Out1) -> Merge/1
  Constant/1 -> If Action Subsystem/1(In1)
  XMV/1 -> If Action Subsystem2/1(In1), If/1

== system mylib/Control valve/Subsystem ==
  XMV(I) : Inport
  "VCV(I) " : Inport  Port=2
  IVST(I) : Inport  Port=3
  If Action Subsystem : Subsystem  TreatAsAtomicUnit=on
  Subsystem : Subsystem
  VCV(I) : Outport  VectorParamsAs1DForOutWhenUnconnected=off
  wires:
  If Action Subsystem/1(VCV(I)) -> VCV(I)/1
  XMV(I)/1 -> Subsystem/1(XMV(I)), If Action Subsystem/1(XMV(I))
  Subsystem/1(if) -> If Action Subsystem/Action
  "VCV(I) "/1 -> Subsystem/2(VCV(I))
  IVST(I)/1 -> Subsystem/3(IVST(I))

== system mylib/Disturbance calculations I=1-9/If Action Subsystem ==
  IDVWLK : Inport
  "DIST " : Inport  Port=2
  G : Inport  Port=3
  Distrubance constants : Inport  Port=4
  Action Port : ActionPort
  Bus Creator : BusCreator  Inputs=6
  Bus Selector : BusSelector  OutputSignals=ADIST,BDIST,CDIST,DDIST,TNEXT,TLAST
  Disturbance parameters I=1-9 : Subsystem
      mask Display:
      | color('Green'), disp('Disturbance parameters\n I=1-9');
      | color('Blue');
      | port_label('input',1,'ADIST');
      | port_label('input',2,'BDIST');
      | port_label('input',3,'CDIST');
      | port_label('input',4,'DDIST');
      | port_label('input',5,'TNEXT');
      | port_label('input',6,'TLAST');
      | port_label('input',7,'IDVWLK');
      | port_label('input',8,'Distrubance constants');
      | port_label('input',9,'G');
      | port_label('output',1,'ADIST');
      | port_label('output',2,'BDIST');
      | port_label('output',3,'CDIST');
      | port_label('output',4,'DDIST');
      | port_label('output',5,'TNEXT');
      | port_label('output',6,'TLAST');
      | port_label('output',7,'G_NEW');
  DIST_NEW : Outport  PortDimensions=6  VectorParamsAs1DForOutWhenUnconnected=off
  G_NEW : Outport  Port=2  OutputWhenDisabled=reset  InitialOutput=0  VectorParamsAs1DForOutWhenUnconnected=off
  wires:
  Disturbance parameters I=1-9/5("TNEXT ") -> Bus Creator/5  "TNEXT"
  Bus Creator/1 -> DIST_NEW/1
  IDVWLK/1 -> Disturbance parameters I=1-9/7(IDVWLK)
  Bus Selector/1 -> Disturbance parameters I=1-9/1(ADIST)  "<ADIST>"
  Distrubance constants/1 -> Disturbance parameters I=1-9/8(Distrubance consatnts)
  Bus Selector/2 -> Disturbance parameters I=1-9/2(BDIST)  "<BDIST>"
  Disturbance parameters I=1-9/1("ADIST ") -> Bus Creator/1  "ADIST"
  Bus Selector/6 -> Disturbance parameters I=1-9/6(TLAST)  "<TLAST>"
  Bus Selector/5 -> Disturbance parameters I=1-9/5(TNEXT)  "<TNEXT>"
  Disturbance parameters I=1-9/4("DDIST ") -> Bus Creator/4  "DDIST"
  Disturbance parameters I=1-9/3("CDIST ") -> Bus Creator/3  "CDIST"
  Bus Selector/4 -> Disturbance parameters I=1-9/4(DDIST)  "<DDIST>"
  Disturbance parameters I=1-9/6("TLAST  ") -> Bus Creator/6  "TLAST"
  Bus Selector/3 -> Disturbance parameters I=1-9/3(CDIST)  "<CDIST>"
  "DIST "/1 -> Bus Selector/1
  Disturbance parameters I=1-9/2("BDIST ") -> Bus Creator/2  "BDIST"
  G/1 -> Disturbance parameters I=1-9/9(G)
  Disturbance parameters I=1-9/7(G_NEW) -> G_NEW/1

== system mylib/Disturbance calculations I=1-9/If Action Subsystem1 ==
  DIST_0 : Inport
  Action Port : ActionPort
  DIST : Outport  VectorParamsAs1DForOutWhenUnconnected=off
  wires:
  DIST_0/1 -> DIST/1

== system mylib/Disturbance calculations I=1-9/Subsystem ==
  TNEXT : Inport
  Clock : Clock
  Constant : Constant  Value=3600
  Data Type Conversion : DataTypeConversion  OutDataTypeStr=double
  If : If  NumInputs=2  IfExpression=u1 == 0  ElseIfExpressions=u1 >= u2  ShowElse=off
  Product : Product
  Product1 : Product  OutDataTypeStr=fixdt(1,32,10)
  if : Outport
  elseif : Outport  Port=2
  wires:
  If/2 -> elseif/1
  If/1 -> if/1
  Constant/1 -> Product1/1, Product/2
  Clock/1 -> Product/1
  Product/1 -> If/1
  TNEXT/1 -> Product1/2
  Product1/1 -> Data Type Conversion/1
  Data Type Conversion/1 -> If/2

== system mylib/Disturbance calculations I=1-9/Subsystem1 ==
  DIST_NEW : Inport
  Bus Creator : BusCreator  Inputs=6
  Bus Selector : BusSelector  OutputSignals=ADIST,BDIST,CDIST,DDIST,TNEXT,TLAST
  Delay{,1..5} (6 alike) : Delay  DelayLength=1  InitialCondition=0
  DIST : Outport
  wires:
  Bus Selector/1 -> Delay/1  "<ADIST>"
  Bus Selector/6 -> Delay5/1  "<TLAST>"
  Delay1/1 -> Bus Creator/2  "BDIST"
  Delay5/1 -> Bus Creator/6  "TLAST"
  Bus Selector/3 -> Delay2/1  "<CDIST>"
  Delay2/1 -> Bus Creator/3  "CDIST"
  Bus Selector/2 -> Delay1/1  "<BDIST>"
  Bus Selector/4 -> Delay3/1  "<DDIST>"
  Delay4/1 -> Bus Creator/5  "TNEXT"
  Bus Selector/5 -> Delay4/1  "<TNEXT>"
  Delay3/1 -> Bus Creator/4  "DDIST"
  Delay/1 -> Bus Creator/1  "ADIST"
  Bus Creator/1 -> DIST/1
  DIST_NEW/1 -> Bus Selector/1

== system mylib/Disturbance calculations I=1-9/Subsystem2 ==
  In2 : Inport
  G : Inport  Port=2
  If Action Subsystem : Subsystem  TreatAsAtomicUnit=on
  If Action Subsystem1 : Subsystem  TreatAsAtomicUnit=on
  If5 : If  IfExpression=u1 == 0
  Merge : Merge
  G1 : Outport  VectorParamsAs1DForOutWhenUnconnected=off
  wires:
  In2/1 -> If Action Subsystem1/1(In1), If5/1
  If5/2 -> If Action Subsystem1/Action
  If Action Subsystem1/1(Out1) -> Merge/1
  If5/1 -> If Action Subsystem/Action
  If Action Subsystem/1(Out1) -> Merge/2
  G/1 -> If Action Subsystem/1(In1)
  Merge/1 -> G1/1

== system mylib/Disturbance parameters I=1-9/Subsystem ==
  TNEXT : Inport
  TLAST : Inport  Port=2
  HWLK : Sum  Inputs=+-
  "HWLK " : Outport  VectorParamsAs1DForOutWhenUnconnected=off
  wires:
  TNEXT/1 -> HWLK/1
  TLAST/1 -> HWLK/2
  HWLK/1 -> "HWLK "/1

== system mylib/Disturbance parameters I=1-9/Subsystem1 ==
  ADIST : Inport
  BDIST : Inport  Port=2
  CDIST : Inport  Port=3
  DDIST : Inport  Port=4
  HWLK : Inport  Port=5
  Add : Sum
  Add1 : Sum
  Product : Product
  Product1 : Product
  Product2 : Product
  SWLK : Sum
  "SWLK " : Outport  VectorParamsAs1DForOutWhenUnconnected=off
  wires:
  BDIST/1 -> Add1/2
  ADIST/1 -> SWLK/1
  CDIST/1 -> Add/2
  SWLK/1 -> "SWLK "/1
  Product/1 -> Add/1
  Add/1 -> Product1/2
  Product2/1 -> SWLK/2
  DDIST/1 -> Product/2
  Product1/1 -> Add1/1
  Add1/1 -> Product2/2
  HWLK/1 -> Product2/1, Product1/1, Product/1

== system mylib/Disturbance parameters I=1-9/Subsystem2 ==
  BDIST : Inport
  CDIST : Inport  Port=2
  DDIST : Inport  Port=3
  HWLK : Inport  Port=4
  Add2 : Sum
  Constant : Constant  Value=3
  Constant1 : Constant  Value=2
  Product3 : Product  Inputs=3
  Product4 : Product
  Product5 : Product
  SPWLK : Sum
  "SPWLK " : Outport  VectorParamsAs1DForOutWhenUnconnected=off
  wires:
  DDIST/1 -> Product3/3
  Product4/1 -> Add2/2
  SPWLK/1 -> "SPWLK "/1
  Add2/1 -> Product5/2
  Constant/1 -> Product3/1
  Product5/1 -> SPWLK/2
  HWLK/1 -> Product5/1, Product3/2
  Product3/1 -> Add2/1
  Constant1/1 -> Product4/1
  CDIST/1 -> Product4/2
  BDIST/1 -> SPWLK/1

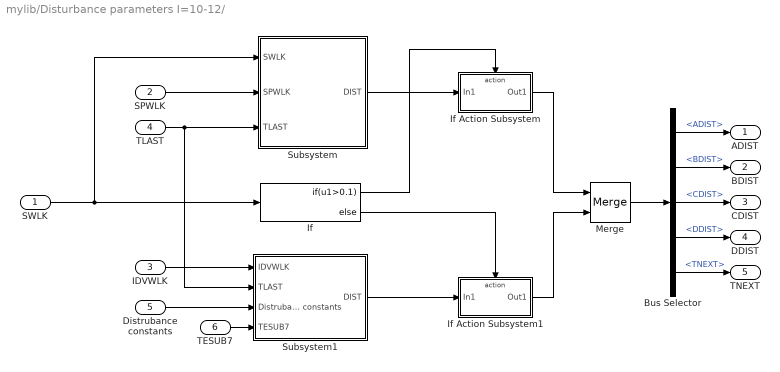
== system mylib/Disturbance parameters I=10-12/  ==
  SWLK : Inport
  SPWLK : Inport  Port=2
  IDVWLK : Inport  Port=3
  TLAST : Inport  Port=4
  Distrubance constants : Inport  Port=5
  TESUB7 : Inport  Port=6
  Bus Selector : BusSelector  OutputSignals=ADIST,BDIST,CDIST,DDIST,TNEXT
  If : If  IfExpression=u1>0.1
  If Action Subsystem : Subsystem  TreatAsAtomicUnit=on
  If Action Subsystem1 : Subsystem  TreatAsAtomicUnit=on
  Merge : Merge
  Subsystem : Subsystem
  Subsystem1 : Subsystem
  ADIST : Outport  VectorParamsAs1DForOutWhenUnconnected=off
  BDIST : Outport  Port=2  VectorParamsAs1DForOutWhenUnconnected=off
  CDIST : Outport  Port=3  VectorParamsAs1DForOutWhenUnconnected=off
  DDIST : Outport  Port=4  VectorParamsAs1DForOutWhenUnconnected=off
  TNEXT : Outport  Port=5  VectorParamsAs1DForOutWhenUnconnected=off
  wires:
  IDVWLK/1 -> Subsystem1/1(IDVWLK)
  SPWLK/1 -> Subsystem/2(SPWLK)
  SWLK/1 -> Subsystem/1(SWLK), If/1
  TLAST/1 -> Subsystem1/2(TLAST), Subsystem/3(TLAST)
  If/1 -> If Action Subsystem/Action
  If/2 -> If Action Subsystem1/Action
  Subsystem1/1(DIST) -> If Action Subsystem1/1(In1)
  Subsystem/1(DIST) -> If Action Subsystem/1(In1)
  If Action Subsystem/1(Out1) -> Merge/1
  If Action Subsystem1/1(Out1) -> Merge/2
  Merge/1 -> Bus Selector/1
  Distrubance constants/1 -> Subsystem1/3(Distrubance constants)
  Bus Selector/1 -> ADIST/1  "<ADIST>"
  Bus Selector/2 -> BDIST/1  "<BDIST>"
  Bus Selector/3 -> CDIST/1  "<CDIST>"
  Bus Selector/4 -> DDIST/1  "<DDIST>"
  Bus Selector/5 -> TNEXT/1  "<TNEXT>"
  TESUB7/1 -> Subsystem1/4(TESUB7)

== system mylib/Disturbance parameters I=10-12/Subsystem ==
  TNEXT : Inport
  TLAST : Inport  Port=2
  HWLK : Sum  Inputs=+-
  "HWLK " : Outport  VectorParamsAs1DForOutWhenUnconnected=off
  wires:
  TNEXT/1 -> HWLK/1
  TLAST/1 -> HWLK/2
  HWLK/1 -> "HWLK "/1

== system mylib/Disturbance parameters I=10-12/Subsystem1 ==
  ADIST : Inport
  BDIST : Inport  Port=2
  CDIST : Inport  Port=3
  DDIST : Inport  Port=4
  HWLK : Inport  Port=5
  Add : Sum
  Add1 : Sum
  Product : Product
  Product1 : Product
  Product2 : Product
  SWLK : Sum
  "SWLK " : Outport  VectorParamsAs1DForOutWhenUnconnected=off
  wires:
  BDIST/1 -> Add1/2
  ADIST/1 -> SWLK/1
  CDIST/1 -> Add/2
  SWLK/1 -> "SWLK "/1
  Product/1 -> Add/1
  Add/1 -> Product1/2
  Product2/1 -> SWLK/2
  DDIST/1 -> Product/2
  Product1/1 -> Add1/1
  Add1/1 -> Product2/2
  HWLK/1 -> Product2/1, Product1/1, Product/1

== system mylib/Disturbance parameters I=10-12/Subsystem2 ==
  BDIST : Inport
  CDIST : Inport  Port=2
  DDIST : Inport  Port=3
  HWLK : Inport  Port=4
  Add2 : Sum
  Constant : Constant  Value=3
  Constant1 : Constant  Value=2
  Product3 : Product  Inputs=3
  Product4 : Product
  Product5 : Product
  SPWLK : Sum
  "SPWLK " : Outport  VectorParamsAs1DForOutWhenUnconnected=off
  wires:
  DDIST/1 -> Product3/3
  Product4/1 -> Add2/2
  SPWLK/1 -> "SPWLK "/1
  Add2/1 -> Product5/2
  Constant/1 -> Product3/1
  Product5/1 -> SPWLK/2
  HWLK/1 -> Product5/1, Product3/2
  Product3/1 -> Add2/1
  Constant1/1 -> Product4/1
  CDIST/1 -> Product4/2
  BDIST/1 -> SPWLK/1

== system mylib/Enthalpy of Stream /Calculate Enthalpy if ITY=2 ==
  T : Inport
  H : Inport  Port=2
  Add : Sum
  Add1 : Sum  Inputs=+-
  Constant : Constant  Value=3.57696
  Constant1 : Constant  Value=1e6
  Constant2 : Constant  Value=273.15
  Divide : Product  Inputs=*/
  Divide1 : Product
  "H " : Outport  VectorParamsAs1DForOutWhenUnconnected=off
  wires:
  T/1 -> Add/1
  Divide1/1 -> Add1/2
  Divide/1 -> Divide1/2
  H/1 -> Add1/1
  Add/1 -> Divide1/1
  Constant2/1 -> Add/2
  Add1/1 -> "H "/1
  Constant/1 -> Divide/1
  Constant1/1 -> Divide/2

== system mylib/Enthalpy of Stream /Calculate Molar Liquid Enthalpy of stream MBtu//lb-mol ==
  T : Inport
  XST(I,1) : Inport  Port=2
  Constant : Constant  Value=XMW
  HI Enthalpy of individual components MBtu/lb : Subsystem
  Product : Product  Inputs=3
  Sum of Elements : Sum  Inputs=+
  H : Outport  VectorParamsAs1DForOutWhenUnconnected=off
  wires:
  Sum of Elements/1 -> H/1
  T/1 -> HI Enthalpy of individual components MBtu/lb/1(T)
  Product/1 -> Sum of Elements/1
  HI Enthalpy of individual components MBtu/lb/1("HI ") -> Product/1
  Constant/1 -> Product/2
  XST(I,1)/1 -> Product/3

== system mylib/Enthalpy of Stream /Calculate Molar Vapour Enthalpy of stream MBtu//lb-mol ==
  T : Inport
  XST(I,1) : Inport  Port=2
  Constant : Constant  Value=XMW
  HI Enthalpy of individual components MBtu/lb : Subsystem
  Product : Product  Inputs=3
  Sum of Elements : Sum  Inputs=+
  H : Outport  VectorParamsAs1DForOutWhenUnconnected=off
  wires:
  Sum of Elements/1 -> H/1
  T/1 -> HI Enthalpy of individual components MBtu/lb/1(T)
  Product/1 -> Sum of Elements/1
  HI Enthalpy of individual components MBtu/lb/1("HI ") -> Product/1
  Constant/1 -> Product/2
  XST(I,1)/1 -> Product/3

== system mylib/Enthalpy of Stream /If Action Subsystem ==
  In1 : Inport
  Action Port : ActionPort
  Out1 : Outport  VectorParamsAs1DForOutWhenUnconnected=off
  wires:
  In1/1 -> Out1/1

== system mylib/Enthalpy of Stream /If Action Subsystem1 ==
  In1 : Inport
  Action Port : ActionPort
  Out1 : Outport  VectorParamsAs1DForOutWhenUnconnected=off
  wires:
  In1/1 -> Out1/1

== system mylib/Enthalpy of Stream /If Action Subsystem2 ==
  In1 : Inport
  Action Port : ActionPort
  Out1 : Outport  VectorParamsAs1DForOutWhenUnconnected=off
  wires:
  In1/1 -> Out1/1

== system mylib/Exergy/Subsystem ==
  ITY : Inport
  "XST " : Inport  Port=2
  If : If  IfExpression=u1 == 0
  If Action Subsystem : Subsystem  TreatAsAtomicUnit=on
  If Action Subsystem1 : $bdroot/Exergy/Subsystem/If Action Subsystem  SystemSampleTime=-1  Latency=0  AutoFrameSizeCalculation=off
  Merge : Merge
  Product1 : Product
  Product2 : Product
  Standard chemical exergy liquid J/mol : Constant  Value=BCHL
  Standard chemical exergy vapour J/mol : Constant  Value=BCHV
  Sum of Elements : Sum  Inputs=+
  Sum of Elements1 : Sum  Inputs=+
  Bch J/mol : Outport  VectorParamsAs1DForOutWhenUnconnected=off
  wires:
  Standard chemical exergy vapour J/mol/1 -> Product1/1
  "XST "/1 -> Product1/2, Product2/2
  Product1/1 -> Sum of Elements/1
  Sum of Elements/1 -> If Action Subsystem1/1
  ITY/1 -> If/1
  Product2/1 -> Sum of Elements1/1
  Standard chemical exergy liquid J/mol/1 -> Product2/1
  Sum of Elements1/1 -> If Action Subsystem/1(In1)
  If/1 -> If Action Subsystem/Action
  If/2 -> If Action Subsystem1/Action
  If Action Subsystem/1(Out1) -> Merge/1
  If Action Subsystem1/1 -> Merge/2
  Merge/1 -> Bch J/mol/1

== system mylib/Exergy/Subsystem2 ==
  ITY : Inport
  Temperature of stream °C : Inport  Port=2
  XST : Inport  Port=3
  P : Inport  Port=4
  Reference Temperature °C : Constant  Value=25
  Subsystem : Subsystem
  Subsystem1 : Subsystem
  Subtract1 : Sum  Inputs=+-
  Bph MBtu/lb-mol : Outport  VectorParamsAs1DForOutWhenUnconnected=off
  wires:
  XST/1 -> Subsystem1/3(XST), Subsystem/3(XST)
  ITY/1 -> Subsystem1/1(ITY), Subsystem/1(ITY)
  Subsystem1/1(T0(s-s0) MBtu/lb-mol) -> Subtract1/2
  Subsystem/1(h-h0 MBtu/lb-mol) -> Subtract1/1
  Temperature of stream °C/1 -> Subsystem1/2(Temperature of stream °C), Subsystem/2(Temperature of stream °C)
  Subtract1/1 -> Bph MBtu/lb-mol/1
  Reference Temperature °C/1 -> Subsystem/4(Reference Temperature), Subsystem1/4(Reference Temperature)
  P/1 -> Subsystem1/5(P)

== system mylib/Exergy Molar Flow/Subsystem ==
  ITY : Inport
  "XST " : Inport  Port=2
  If : If  IfExpression=u1 == 0
  If Action Subsystem : Subsystem  TreatAsAtomicUnit=on
  If Action Subsystem1 : $bdroot/Exergy/Subsystem/If Action Subsystem  SystemSampleTime=-1  Latency=0  AutoFrameSizeCalculation=off
  Merge : Merge
  Product1 : Product
  Product2 : Product
  Standard chemical exergy liquid kJ/mol : Constant  Value=BCHL
  Standard chemical exergy vapour kJ/mol : Constant  Value=BCHV
  Sum of Elements : Sum  Inputs=+
  Sum of Elements1 : Sum  Inputs=+
  Bch kJ/mol : Outport  VectorParamsAs1DForOutWhenUnconnected=off
  wires:
  Merge/1 -> Bch kJ/mol/1
  If Action Subsystem1/1 -> Merge/2
  If Action Subsystem/1(Out1) -> Merge/1
  If/2 -> If Action Subsystem1/Action
  If/1 -> If Action Subsystem/Action
  Sum of Elements1/1 -> If Action Subsystem/1(In1)
  Standard chemical exergy liquid kJ/mol/1 -> Product2/1
  Product2/1 -> Sum of Elements1/1
  ITY/1 -> If/1
  Sum of Elements/1 -> If Action Subsystem1/1
  Product1/1 -> Sum of Elements/1
  "XST "/1 -> Product2/2, Product1/2
  Standard chemical exergy vapour kJ/mol/1 -> Product1/1

== system mylib/Exergy Molar Flow/Subsystem2 ==
  ITY : Inport
  Temperature of stream °C : Inport  Port=2
  XST : Inport  Port=3
  P : Inport  Port=4
  Reference Temperature °C : Constant  Value=25
  Subsystem : Subsystem
  Subsystem1 : Subsystem
  Subtract1 : Sum  Inputs=+-
  Bph MBtu/lb-mol : Outport  VectorParamsAs1DForOutWhenUnconnected=off
  wires:
  P/1 -> Subsystem1/5(P)
  Reference Temperature °C/1 -> Subsystem1/4(Reference Temperature), Subsystem/4(Reference Temperature)
  Subtract1/1 -> Bph MBtu/lb-mol/1
  Temperature of stream °C/1 -> Subsystem/2(Temperature of stream °C), Subsystem1/2(Temperature of stream °C)
  Subsystem/1(h-h0 MBtu/lb-mol) -> Subtract1/1
  Subsystem1/1(T0(s-s0) MBtu/lb-mol) -> Subtract1/2
  ITY/1 -> Subsystem/1(ITY), Subsystem1/1(ITY)
  XST/1 -> Subsystem/3(XST), Subsystem1/3(XST)

== system mylib/Integration/Subsystem ==
  In1 : Inport
  Clock : Clock
  If : If  NumInputs=2  IfExpression=u1 > 0 & u2~=0
  If Action Subsystem : Subsystem  TreatAsAtomicUnit=on
  If Action Subsystem1 : Subsystem  TreatAsAtomicUnit=on
  Merge : Merge
  Out1 : Outport
  wires:
  If Action Subsystem/1(Out1) -> Merge/1
  Clock/1 -> If/1
  If/2 -> If Action Subsystem1/Action
  If/1 -> If Action Subsystem/Action
  If Action Subsystem1/1(Out1) -> Merge/2
  [ISD] -> If/2
  In1/1 -> If Action Subsystem1/1(In1)
  Merge/1 -> Out1/1
